simulink model "Torque_regulation_22b"  (R2022b)
settings: Solver=FixedStepAuto  StartTime=0.0  StopTime=20  RelTol=1e-3
settings Model: Creator=akame  LastModifiedBy=jungi
settings OptimizationCC: DefaultParameterBehavior=Inlined  UseDivisionForNetSlopeComputation=on  GainParamInheritBuiltInType=on  UseFloatMulNetSlope=on  InlineInvariantSignals=on  ReuseModelBlockBuffer=on  PassReuseOutputArgsAs=Individual arguments  ZeroExternalMemoryAtStartup=off  ZeroInternalMemoryAtStartup=off  NoFixptDivByZeroProtection=on  EfficientFloat2IntCast=on  LifeSpan=1  OptimizeBlockOrder=speed  DifferentSizesBufferReuse=on  EfficientTunableParamExpr=on
settings DebuggingCC: ParameterTunabilityLossMsg=error  SFUnexpectedBacktrackingDiag=warning  SFNoUnconditionalDefaultTransitionDiag=warning
settings HardwareCC: ProdBitPerLong=64  ProdLongLongMode=on  ProdHWDeviceType=Apple->ARM64
settings SFSimCC: MATLABDynamicMemAlloc=off
settings RTWCC: Description=Embedded Coder  SystemTargetFile=ert.tlc  TemplateMakefile=ert_default_tmf  GenerateReport=on  BuildConfiguration=Debug  LaunchReport=on  TargetLang=C++  GPUComputeCapability=5.0
settings CodeAppCC: ForceParamTrailComments=on  IgnoreCustomStorageClasses=off  OperatorAnnotations=on  SimulinkDataObjDesc=on  SFDataObjDesc=on  CustomSymbolStrGlobalVar=rt$N$M  CustomSymbolStrType=$N$M  CustomSymbolStrFcn=$N$M$F  CustomSymbolStrMacro=$N$M  InsertBlockDesc=on  EnableCustomComments=on
settings ERTTargetCC: TargetLangStandard=C++11 (ISO)  GenerateSampleERTMain=on  IncludeMdlTerminateFcn=off  CombineSignalStateStructs=on  CodeInterfacePackaging=C++ class  SupportComplex=off  SupportContinuousTime=on  InlinedParameterPlacement=NonHierarchical  RootIOFormat=Structure reference  ERTCustomFileTemplate=example_file_process.tlc  ERTFilePackagingFormat=CompactWithDataFile
settings ConfigComp: CovBoundaryAbsTol=1.0e-5

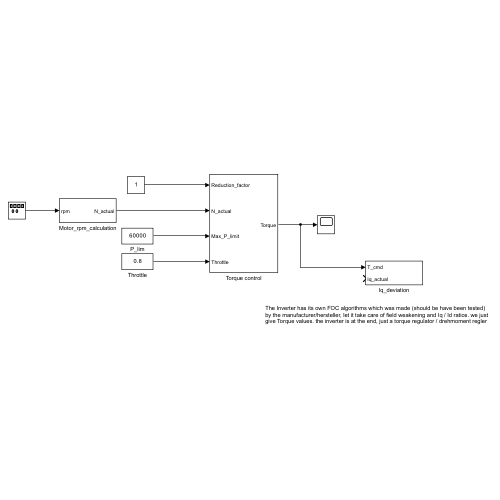
[thumbnail: Simulink's stored preview of the top-level diagram]
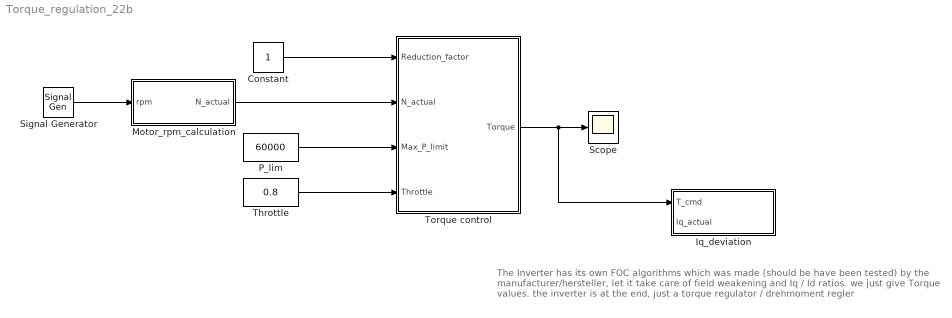
== system Torque_regulation_22b ==
  note: The Inverter has its own FOC algorithms which was made (should be have been tested) by the manufacturer/hersteller, let it take care of field weakening and Iq / Id ratios. we just give Torque values. the inverter is at the end, just a torque regulator / drehmoment regler
  Constant : Constant
  Iq_deviation : Subsystem
  Motor_rpm_calculation : Subsystem
  P_lim : Constant  Value=60000
  Scope : Scope
  Signal Generator : SignalGenerator  Amplitude=2000  Frequency=0.5  Units=rad/sec
  Throttle : Constant  Value=0.8
  Torque control : Subsystem
  wires:
  Constant/1 -> Torque control/1(Reduction_factor)
  Signal Generator/1 -> Motor_rpm_calculation/1(rpm)
  Throttle/1 -> Torque control/4(Throttle)
  P_lim/1 -> Torque control/3(Max_P_limit)
  Torque control/1(Torque) -> Iq_deviation/1(T_cmd), Scope/1
  Motor_rpm_calculation/1(N_actual) -> Torque control/2(N_actual)

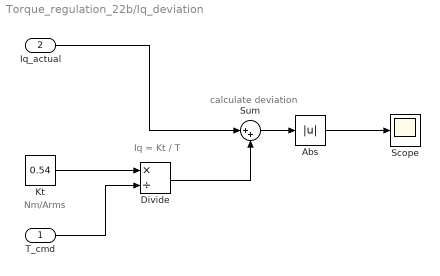
== system Torque_regulation_22b/Iq_deviation ==
  note: calculate deviation
  note: Iq = Kt / T
  note: Nm/Arms
  T_cmd : Inport
  Iq_actual : Inport  Port=2
  Abs : Abs  SaturateOnIntegerOverflow=off
  Divide : Product  Inputs=*/
  Kt : Constant  Value=0.54
  Scope : Scope
  Sum : Sum  Inputs=|++
  wires:
  Kt/1 -> Divide/1
  T_cmd/1 -> Divide/2
  Iq_actual/1 -> Sum/1
  Divide/1 -> Sum/2
  Sum/1 -> Abs/1
  Abs/1 -> Scope/1

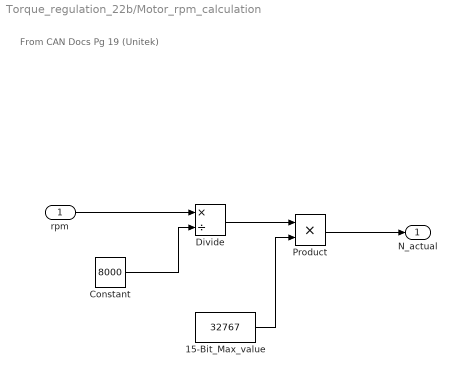
== system Torque_regulation_22b/Motor_rpm_calculation ==
  note: From CAN Docs Pg 19
      | (Unitek)
  rpm : Inport
  15-Bit_Max_value : Constant  Value=32767
  Constant : Constant  Value=8000
  Divide : Product  Inputs=*/
  Product : Product
  N_actual : Outport
  wires:
  rpm/1 -> Divide/1
  Divide/1 -> Product/1
  15-Bit_Max_value/1 -> Product/2
  Constant/1 -> Divide/2
  Product/1 -> N_actual/1

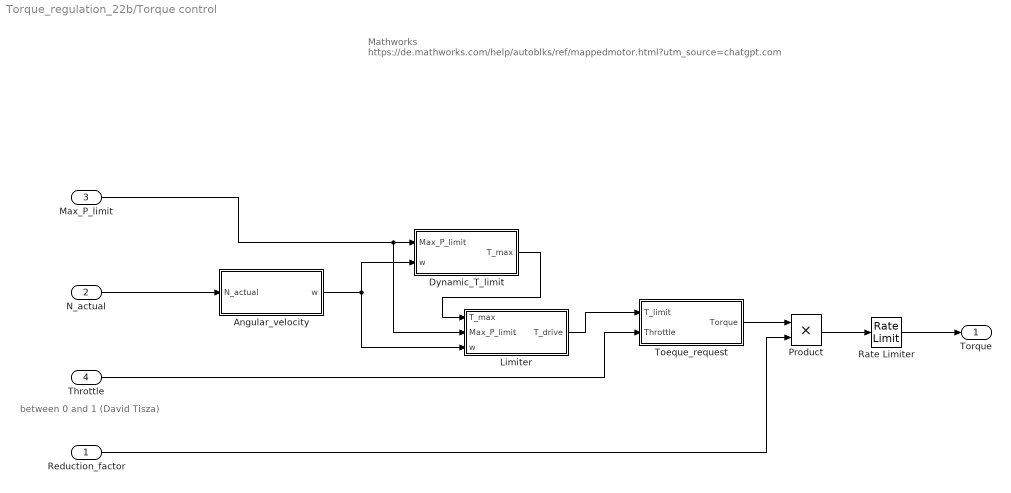
== system Torque_regulation_22b/Torque control ==
  note: between 0 and 1 (David Tisza)
  note: Mathworks
      | https://de.mathworks.com/help/autoblks/ref/mappedmotor.html?utm_source=chatgpt.com
  Reduction_factor : Inport
  N_actual : Inport  Port=2
  Max_P_limit : Inport  Port=3
  Throttle : Inport  Port=4
  Angular_velocity : Subsystem
  Dynamic_T_limit : Subsystem
  Limiter : Subsystem
  Product : Product
  Rate Limiter : RateLimiter  SampleTimeMode=inherited
  Toeque_request : Subsystem
  Torque : Outport
  wires:
  N_actual/1 -> Angular_velocity/1(N_actual)
  Throttle/1 -> Toeque_request/2(Throttle)
  Angular_velocity/1(w) -> Dynamic_T_limit/2(w), Limiter/3(w)
  Max_P_limit/1 -> Limiter/2(Max_P_limit), Dynamic_T_limit/1(Max_P_limit)
  Dynamic_T_limit/1(T_max) -> Limiter/1(T_max)
  Limiter/1(T_drive) -> Toeque_request/1(T_limit)
  Toeque_request/1(Torque) -> Product/1
  Rate Limiter/1 -> Torque/1
  Reduction_factor/1 -> Product/2
  Product/1 -> Rate Limiter/1

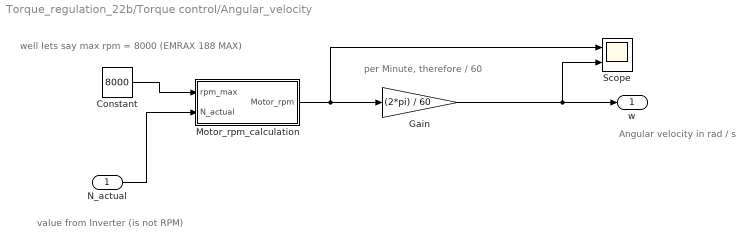
== system Torque_regulation_22b/Torque control/Angular_velocity ==
  note: Angular velocity in
      | rad / s
  note: per Minute, therefore / 60
  note: value from Inverter (is not RPM)
  note: well lets say max rpm = 8000 (EMRAX 188 MAX)
  N_actual : Inport
  Constant : Constant  Value=8000
  Gain : Gain  Gain=(2*pi) / 60
  Motor_rpm_calculation : Subsystem
  Scope : Scope  NumInputPorts=2
  w : Outport
  wires:
  N_actual/1 -> Motor_rpm_calculation/2(N_actual)
  Constant/1 -> Motor_rpm_calculation/1(rpm_max)
  Gain/1 -> Scope/2, w/1
  Motor_rpm_calculation/1(Motor_rpm) -> Scope/1, Gain/1

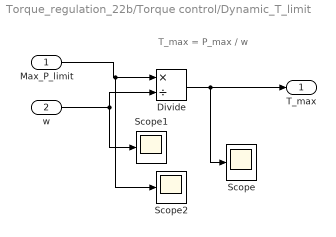
== system Torque_regulation_22b/Torque control/Dynamic_T_limit ==
  note: T_max = P_max / w
  Max_P_limit : Inport
  w : Inport  Port=2
  Divide : Product  Inputs=*/
  Scope : Scope
  Scope1 : Scope
  Scope2 : Scope
  T_max : Outport
  wires:
  w/1 -> Scope1/1, Divide/2
  Max_P_limit/1 -> Scope2/1, Divide/1
  Divide/1 -> Scope/1, T_max/1

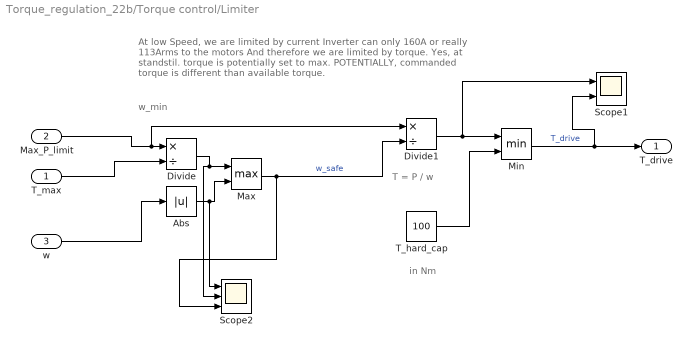
== system Torque_regulation_22b/Torque control/Limiter ==
  note: T = P / w
  note: in Nm
  note: At low Speed, we are limited by current
      | Inverter can only 160A or really 113Arms to the motors
      |
      | And therefore we are limited by torque.
      | Yes, at standstil. torque is potentially set to max.
      | POTENTIALLY, commanded torque is different than available torque.
  note: w_min
  T_max : Inport
  Max_P_limit : Inport  Port=2
  w : Inport  Port=3
  Abs : Abs  SaturateOnIntegerOverflow=off
  Divide : Product  Inputs=*/
  Divide1 : Product  Inputs=*/
  Max : MinMax  Function=max  Inputs=2
  Min : MinMax  Inputs=2
  Scope1 : Scope  NumInputPorts=2
  Scope2 : Scope  NumInputPorts=3
  T_hard_cap : Constant  Value=100
  T_drive : Outport
  wires:
  Max_P_limit/1 -> Divide1/1, Divide/1
  T_max/1 -> Divide/2
  w/1 -> Abs/1
  Divide/1 -> Max/1, Scope2/2
  Abs/1 -> Scope2/1, Max/2
  Max/1 -> Divide1/2, Scope2/3  "w_safe"
  Divide1/1 -> Scope1/1, Min/1
  T_hard_cap/1 -> Min/2
  Min/1 -> Scope1/2, T_drive/1  "T_drive"

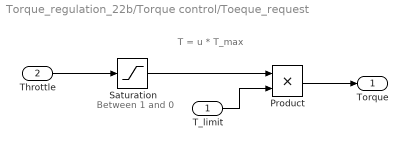
== system Torque_regulation_22b/Torque control/Toeque_request ==
  note: T = u * T_max
  note: Between 1 and 0
  T_limit : Inport
  Throttle : Inport  Port=2
  Product : Product
  Saturation : Saturate  UpperLimit=1  LowerLimit=0
  Torque : Outport
  wires:
  Throttle/1 -> Saturation/1
  Saturation/1 -> Product/1
  T_limit/1 -> Product/2
  Product/1 -> Torque/1

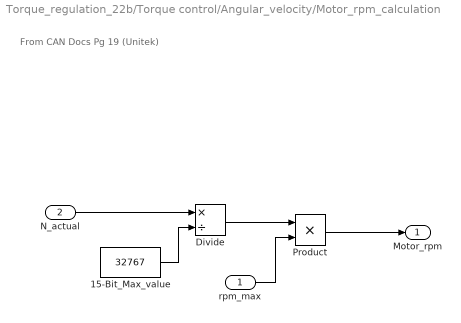
== system Torque_regulation_22b/Torque control/Angular_velocity/Motor_rpm_calculation ==
  note: From CAN Docs Pg 19
      | (Unitek)
  rpm_max : Inport
  N_actual : Inport  Port=2
  15-Bit_Max_value : Constant  Value=32767
  Divide : Product  Inputs=*/
  Product : Product
  Motor_rpm : Outport
  wires:
  N_actual/1 -> Divide/1
  Divide/1 -> Product/1
  15-Bit_Max_value/1 -> Divide/2
  rpm_max/1 -> Product/2
  Product/1 -> Motor_rpm/1
